simulink model "UGV"  (R2016b)
settings: Solver=VariableStepAuto  StartTime=0.0  StopTime=20  RelTol=1e-3
undefined symbols (not defined in the file or in its folder): UGV_init
settings Model: Creator=nagym  LastModifiedBy=Misi
settings DataIOCC: ReturnWorkspaceOutputs=on
settings SFSimCC: SimUseLocalCustomCode=on
settings RTWCC: RTWUseLocalCustomCode=on

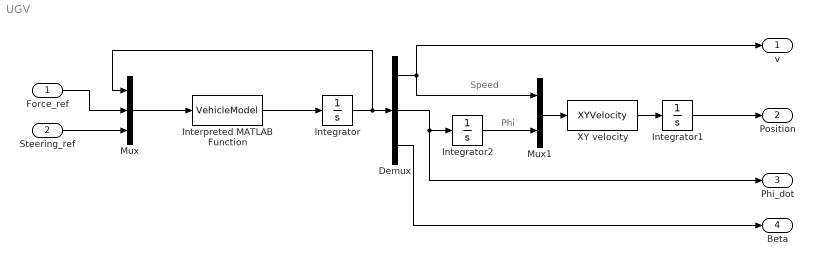
== system UGV ==
  note: Phi
  note: Speed
  Force_ref : Inport
  Steering_ref : Inport  Port=2
  Demux : Demux  Outputs=3
  Integrator : Integrator  InitialCondition=UGV_init
  Integrator1 : Integrator  InitialCondition=[0 0]
  Integrator2 : Integrator  InitialCondition=[1 0 0]
  Interpreted MATLAB Function : MATLABFcn  MATLABFcn=VehicleModel  OutputDimensions=3
  Mux : Mux  Inputs=3
  Mux1 : Mux  Inputs=2
  XY velocity : MATLABFcn  MATLABFcn=XYVelocity  OutputDimensions=2
  v : Outport
  Position : Outport  Port=2
  Phi_dot : Outport  Port=3
  Beta : Outport  Port=4
  wires:
  Integrator/1 -> Demux/1, Mux/1
  Interpreted MATLAB Function/1 -> Integrator/1
  Mux/1 -> Interpreted MATLAB Function/1
  Demux/1 -> Mux1/1, v/1
  Integrator2/1 -> Mux1/2
  Demux/2 -> Phi_dot/1, Integrator2/1
  XY velocity/1 -> Integrator1/1
  Force_ref/1 -> Mux/2
  Steering_ref/1 -> Mux/3
  Mux1/1 -> XY velocity/1
  Demux/3 -> Beta/1
  Integrator1/1 -> Position/1
